simulink model "Simulink_exam"  (R2023a)
settings: Solver=VariableStepAuto  StartTime=0.0  StopTime=30.0  RelTol=1e-3
settings Model: Creator=Simone  LastModifiedBy=Simone

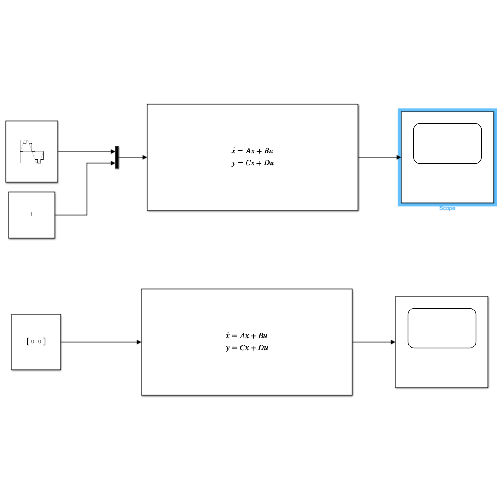
[thumbnail: Simulink's stored preview of the top-level diagram]
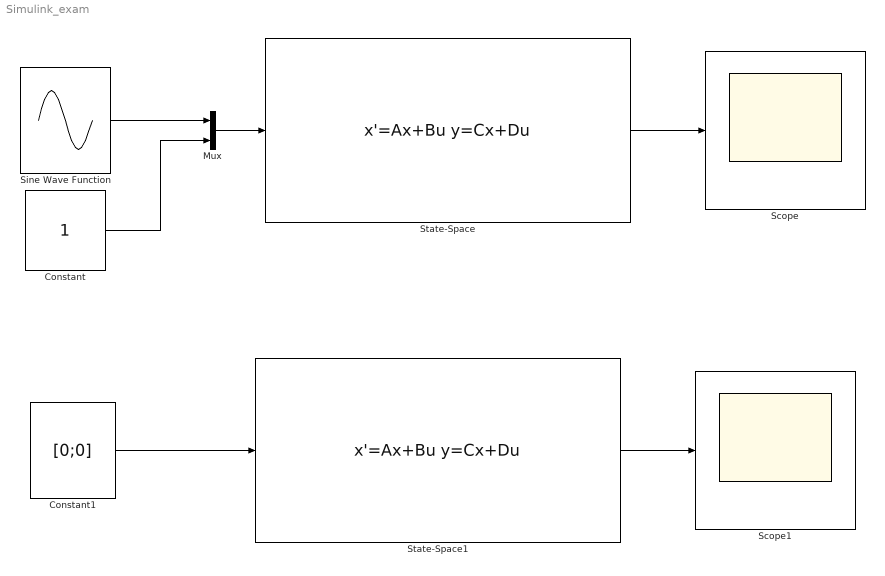
== system Simulink_exam ==
  Constant : Constant
  Constant1 : Constant  Value=[0;0]
  Mux : Mux  Inputs=2
  Scope : Scope
  Scope1 : Scope
  Sine Wave Function : Sin  Amplitude=2  Frequency=3  SampleTime=0.1
  State-Space : StateSpace  A=[-0.5 0 1; 0 -2 0.2; 0 -0.2 -2]  B=[1 0; 0 0; -1 1]  C=[1 0 0; 0 1 -1]  D=[0 0; 0 0]  InitialCondition=[0; 0; 0]
  State-Space1 : StateSpace  A=[-0.5 0 1; 0 -2 0.2; 0 -0.2 -2]  B=[1 0; 0 0; -1 1]  C=[1 0 0; 0 1 -1]  D=[0 0; 0 0]  InitialCondition=[1; 0;1]
  wires:
  State-Space/1 -> Scope/1
  Mux/1 -> State-Space/1
  Sine Wave Function/1 -> Mux/1
  Constant/1 -> Mux/2
  State-Space1/1 -> Scope1/1
  Constant1/1 -> State-Space1/1
